simulink library "adeye_lib"  (R2019a)
settings: Solver=VariableStepAuto  StartTime=0.0  StopTime=10.0  RelTol=1e-3
undefined symbols (not defined in the file): AngularVelocity, Clock_, Data, Data_SL_Info, DiscIntNeverNeededParam, Encoding, Encoding_SL_Info, Header, Height, LinearAcceleration, Orientation, Pose, Step, Twist, Width
libraries: robotlib x47, $bdroot x46, simulink_extras x12, dspsrcs4 x6, dspindex x6, robotcorelib x2, aerolibutil x2, PreScanSimulinkLibrary x1
(part 3 of 4)

== system adeye_lib/ROS Send Camera TL ==
  note: Because the image is RGB
  In1 : Inport
  In2 : Inport  Port=2
  In3 : Inport  Port=3
  Enable : EnablePort
  Assignment2 : Assignment  OutputInitialize=Specify size for each dimension in table  DiagnosticForDimensions=Warning  IndexOptions=Starting index (dialog)  Indices=1  OutputSizes=1000
  Blank Message3 : robotlib/Blank Message  messageClass=Message  entityType=sensor_msgs/Image  messageType=sensor_msgs/Image  SampleTime=inf
      settings: SourceProductBaseCode=RO
  Bus Assignment3 : BusAssignment  AssignedSignals=Height,Width,Encoding,Encoding_SL_Info.CurrentLength,Step,Data,Data_SL_Info.CurrentLength,Header.FrameId,Header.FrameId_SL_Info.CurrentLength
  Bus Selector2 : BusSelector  OutputSignals=Header.FrameId
  Constant19 : Constant  Value=uint8(['rgb8'])
  Constant20 : Constant  Value=uint8(['tl_camera'])
  Constant25 : Constant  Value=3  OutDataTypeStr=Inherit: Inherit via back propagation
  Data Type Conversion1 : DataTypeConversion  OutDataTypeStr=uint8
  Ground_1 : Ground
  Ground_2 : Ground
  Ground_3 : Ground
  Math Function{,1..3} (4 alike) : Math  Operator=transpose  SaturateOnIntegerOverflow=on
  Matrix Concatenate : Concatenate  NumInputs=3  Mode=Multidimensional array  ConcatenateDimension=2
  Product : Product  OutDataTypeStr=uint32
  Publish1 : robotlib/Publish  topicSource=Specify your own  topic=sensor/tl/image_raw  messageType=sensor_msgs/Image  messageQueueLength=1
      settings: SourceProductBaseCode=RO
  Reshape{1,17..19} (4 alike) : Reshape
  Terminator_1 : Terminator
  VECTORES : MATLAB Function  TreatAsAtomicUnit=on
  Variable Selector : dspindex/Variable Selector  NumInputs=1  rowsOrCols=Rows  IdxMode=Fixed  Elements=[1]  ZerOneIdxMode=One-based  errmode=Clip Index  FillMode=on  FillValues=0
  Variable Selector1 : dspindex/Variable Selector  NumInputs=1  rowsOrCols=Rows  IdxMode=Fixed  Elements=[1]  ZerOneIdxMode=One-based  errmode=Clip Index  FillMode=on  FillValues=0
  Width : Width
  Width1 : Width
  Width10 : Width  DataType=uint32
  Width5 : Width  DataType=uint32
  Width9 : Width  DataType=uint32
  wires:
  Reshape19/1 -> Matrix Concatenate/3
  Data Type Conversion1/1 -> Width9/1, Bus Assignment3/7
  Math Function/1 -> Variable Selector/1, Reshape17/1
  Constant25/1 -> Product/2
  Width/1 -> Bus Assignment3/2
  Width9/1 -> Bus Assignment3/8
  Bus Selector2/1 -> Assignment2/1  "<FrameId>"
  Product/1 -> Bus Assignment3/6
  Assignment2/1 -> Bus Assignment3/9
  Bus Assignment3/1 -> Publish1/1
  Constant19/1 -> Width5/1, Bus Assignment3/4
  Reshape18/1 -> Matrix Concatenate/2
  Width5/1 -> Bus Assignment3/5
  Reshape17/1 -> Matrix Concatenate/1
  Width10/1 -> Bus Assignment3/10
  Math Function2/1 -> Reshape19/1
  Constant20/1 -> Assignment2/2, Width10/1
  Width1/1 -> Bus Assignment3/3, Product/1
  Math Function1/1 -> Reshape18/1
  Blank Message3/1 -> Bus Selector2/1, Bus Assignment3/1
  In3/1 -> Math Function2/1
  In2/1 -> Math Function1/1
  In1/1 -> Variable Selector1/1, Math Function/1
  Reshape1/1 -> Data Type Conversion1/1
  Matrix Concatenate/1 -> Math Function3/1
  Math Function3/1 -> Reshape1/1
  Variable Selector/1 -> Width/1
  Variable Selector1/1 -> Width1/1
  Ground_1/1 -> VECTORES/1(imgR)
  Ground_2/1 -> VECTORES/2(imgG)
  Ground_3/1 -> VECTORES/3(imgB)
  VECTORES/1(data) -> Terminator_1/1

== system adeye_lib/ROS Send Clock ==
  note: Nanoseconds
  In1 : Inport
  Enable : EnablePort
  Blank Message3 : robotlib/Blank Message  messageClass=Message  entityType=rosgraph_msgs/Clock  messageType=rosgraph_msgs/Clock  SampleTime=inf
      settings: SourceProductBaseCode=RO
  Bus Assignment : BusAssignment  AssignedSignals=Clock_.Sec,Clock_.Nsec
  Constant2 : Constant  Value=1000000000
  Floor : Rounding  Operator=fix
  Product : Product
  Publish3 : robotlib/Publish  topicSource=Specify your own  topic=/clock  messageType=rosgraph_msgs/Clock  messageQueueLength=1
      settings: SourceProductBaseCode=RO
  Subtract : Sum  Inputs=+-
  wires:
  In1/1 -> Subtract/1, Floor/1
  Floor/1 -> Subtract/2, Bus Assignment/2
  Blank Message3/1 -> Bus Assignment/1
  Bus Assignment/1 -> Publish3/1
  Subtract/1 -> Product/1
  Product/1 -> Bus Assignment/3
  Constant2/1 -> Product/2

== system adeye_lib/ROS Send GNSS ==
  In1 : Inport
  Enable : EnablePort
  Add5 : Sum
  Assignment2 : Assignment  OutputInitialize=Specify size for each dimension in table  DiagnosticForDimensions=Warning  IndexOptions=Starting index (dialog)  Indices=1  OutputSizes=1000
  Blank Message4 : robotlib/Blank Message  messageClass=Message  entityType=geometry_msgs/PoseStamped  messageType=geometry_msgs/PoseStamped  SampleTime=inf
      settings: SourceProductBaseCode=RO
  Bus Assignment3 : BusAssignment  AssignedSignals=Header.Seq,Header.FrameId,Header.FrameId_SL_Info.CurrentLength,Header.Stamp.Sec,Header.Stamp.Nsec,Pose.Position.X,Pose.Position.Y,Pose.Position.Z,Pose.Orientation.W,Pose.Orientation.X,Pose.Orientation.Y,Pose.Orientation.Z
  Bus Selector2 : BusSelector  OutputSignals=Header.FrameId
  Clock : Clock
  Constant24 : Constant  OutDataTypeStr=uint32
  Constant25 : Constant  Value=uint8(['map'])
  Demux : Demux  Outputs=7
  Floor : Rounding  Operator=fix
  Memory2 : Memory  InheritSampleTime=on
  Nanoseconds : Constant  Value=1000000000
  Product : Product
  Publish2 : robotlib/Publish  topicSource=Specify your own  topic=/sensor/gnss_pose  messageType=geometry_msgs/PoseStamped  messageQueueLength=1
      settings: SourceProductBaseCode=RO
  Subtract : Sum  Inputs=+-
  Width5 : Width  DataType=uint32
  wires:
  Bus Assignment3/1 -> Publish2/1
  Demux/5 -> Bus Assignment3/11
  Demux/3 -> Bus Assignment3/9
  Product/1 -> Bus Assignment3/6
  Demux/1 -> Bus Assignment3/7
  Add5/1 -> Memory2/1, Bus Assignment3/2
  Clock/1 -> Subtract/1, Floor/1
  In1/1 -> Demux/1  "pose"
  Assignment2/1 -> Bus Assignment3/3
  Bus Selector2/1 -> Assignment2/1  "<FrameId>"
  Constant24/1 -> Add5/2
  Demux/7 -> Bus Assignment3/13
  Demux/6 -> Bus Assignment3/12
  Constant25/1 -> Width5/1, Assignment2/2
  Nanoseconds/1 -> Product/2
  Memory2/1 -> Add5/1
  Blank Message4/1 -> Bus Selector2/1, Bus Assignment3/1
  Floor/1 -> Bus Assignment3/5, Subtract/2
  Width5/1 -> Bus Assignment3/4
  Demux/2 -> Bus Assignment3/8
  Demux/4 -> Bus Assignment3/10
  Subtract/1 -> Product/1

== system adeye_lib/ROS Send Goal ==
  In1 : Inport
  In2 : Inport  Port=2
  In3 : Inport  Port=3
  In4 : Inport  Port=4
  In5 : Inport  Port=5
  In6 : Inport  Port=6
  In7 : Inport  Port=7
  Enable : EnablePort
  Add4 : Sum
  Assignment4 : Assignment  OutputInitialize=Specify size for each dimension in table  DiagnosticForDimensions=Warning  IndexOptions=Starting index (dialog)  Indices=1  OutputSizes=1000
  Blank Message5 : robotlib/Blank Message  messageClass=Message  entityType=geometry_msgs/PoseStamped  messageType=geometry_msgs/PoseStamped  SampleTime=inf
      settings: SourceProductBaseCode=RO
  Bus Assignment4 : BusAssignment  AssignedSignals=Header.Seq,Header.FrameId,Header.FrameId_SL_Info.CurrentLength,Pose.Position.X,Pose.Position.Y,Pose.Position.Z,Pose.Orientation.W,Pose.Orientation.X,Pose.Orientation.Y,Pose.Orientation.Z
  Bus Selector3 : BusSelector  OutputSignals=Header.FrameId
  Constant8 : Constant  OutDataTypeStr=uint32
  Constant9 : Constant  Value=uint8(['world'])
  Memory1 : Memory  InheritSampleTime=on
  Publish1 : robotlib/Publish  topicSource=Select from ROS network  topic=/move_base_simple/goal  messageType=geometry_msgs/PoseStamped  messageQueueLength=1
      settings: SourceProductBaseCode=RO
  Width4 : Width  DataType=uint32
  wires:
  Blank Message5/1 -> Bus Selector3/1, Bus Assignment4/1
  Add4/1 -> Bus Assignment4/2, Memory1/1
  Assignment4/1 -> Bus Assignment4/3
  Bus Selector3/1 -> Assignment4/1  "<FrameId>"
  Bus Assignment4/1 -> Publish1/1
  Constant8/1 -> Add4/2
  Constant9/1 -> Assignment4/2, Width4/1
  Memory1/1 -> Add4/1
  Width4/1 -> Bus Assignment4/4
  In1/1 -> Bus Assignment4/5
  In2/1 -> Bus Assignment4/6
  In3/1 -> Bus Assignment4/7
  In4/1 -> Bus Assignment4/8
  In5/1 -> Bus Assignment4/9
  In6/1 -> Bus Assignment4/10
  In7/1 -> Bus Assignment4/11

== system adeye_lib/ROS Send Groud Truth Pose ==
  In1 : Inport
  Enable : EnablePort
  Add5 : Sum
  Assignment2 : Assignment  OutputInitialize=Specify size for each dimension in table  DiagnosticForDimensions=Warning  IndexOptions=Starting index (dialog)  Indices=1  OutputSizes=1000
  Blank Message4 : robotlib/Blank Message  messageClass=Message  entityType=geometry_msgs/PoseStamped  messageType=geometry_msgs/PoseStamped  SampleTime=inf
      settings: SourceProductBaseCode=RO
  Bus Assignment3 : BusAssignment  AssignedSignals=Header.Seq,Header.FrameId,Header.FrameId_SL_Info.CurrentLength,Header.Stamp.Sec,Header.Stamp.Nsec,Pose.Position.X,Pose.Position.Y,Pose.Position.Z,Pose.Orientation.W,Pose.Orientation.X,Pose.Orientation.Y,Pose.Orientation.Z
  Bus Selector2 : BusSelector  OutputSignals=Header.FrameId
  Clock : Clock
  Constant24 : Constant  OutDataTypeStr=uint32
  Constant25 : Constant  Value=uint8(['map'])
  Demux : Demux  Outputs=7
  Floor : Rounding  Operator=fix
  Memory2 : Memory  InheritSampleTime=on
  Nanoseconds : Constant  Value=1000000000
  Product : Product
  Publish2 : robotlib/Publish  topicSource=Specify your own  topic=/ground_truth_pose  messageType=geometry_msgs/PoseStamped  messageQueueLength=1
      settings: SourceProductBaseCode=RO
  Subtract : Sum  Inputs=+-
  Width5 : Width  DataType=uint32
  wires:
  Constant25/1 -> Width5/1, Assignment2/2
  Clock/1 -> Subtract/1, Floor/1
  Nanoseconds/1 -> Product/2
  Floor/1 -> Bus Assignment3/5, Subtract/2
  Assignment2/1 -> Bus Assignment3/3
  Bus Assignment3/1 -> Publish2/1
  Blank Message4/1 -> Bus Selector2/1, Bus Assignment3/1
  Demux/4 -> Bus Assignment3/10
  Demux/7 -> Bus Assignment3/13
  Demux/5 -> Bus Assignment3/11
  Width5/1 -> Bus Assignment3/4
  Demux/6 -> Bus Assignment3/12
  Demux/2 -> Bus Assignment3/8
  Product/1 -> Bus Assignment3/6
  In1/1 -> Demux/1  "pose"
  Constant24/1 -> Add5/2
  Bus Selector2/1 -> Assignment2/1  "<FrameId>"
  Add5/1 -> Memory2/1, Bus Assignment3/2
  Subtract/1 -> Product/1
  Memory2/1 -> Add5/1
  Demux/1 -> Bus Assignment3/7
  Demux/3 -> Bus Assignment3/9

== system adeye_lib/ROS Send IMU ==
  In1 : Inport
  In2 : Inport  Port=2
  In3 : Inport  Port=3
  Yaw rate [deg/s] : Inport  Port=4
  Velocity [m/s] : Inport  Port=5
  Enable : EnablePort
  Add5 : Sum
  Assignment2 : Assignment  OutputInitialize=Specify size for each dimension in table  DiagnosticForDimensions=Warning  IndexOptions=Starting index (dialog)  Indices=1  OutputSizes=1000
  Blank Message9 : robotlib/Blank Message  messageClass=Message  entityType=sensor_msgs/Imu  messageType=sensor_msgs/Imu  SampleTime=inf
      settings: SourceProductBaseCode=RO
  Bus Assignment7 : BusAssignment  AssignedSignals=Orientation.W,Orientation.X,Orientation.Y,Orientation.Z,AngularVelocity.Z,LinearAcceleration.X,LinearAcceleration.Z,Header.Seq,Header.FrameId,Header.FrameId_SL_Info.CurrentLength
  Bus Selector2 : BusSelector  OutputSignals=Header.FrameId
  Constant : Constant  Value=-9.82
  Constant1 : Constant  Value=-1
  Constant24 : Constant  OutDataTypeStr=uint32
  Constant25 : Constant  Value=uint8(['velodyne'])
  Coordinate Transformation Conversion : robotcorelib/Coordinate Transformation Conversion  InputRepresentation=Euler Angles  InputEulerSequence=XYZ  ShowTrVecInputPort=on  OutputRepresentation=Quaternion  OutputEulerSequence=ZYX  ShowTrVecOutputPort=on  SimulateUsing=Interpreted execution
      settings: SourceProductBaseCode=RO
  Degrees to Radians{1..4} (4 alike) : simulink_extras/Transformations/Degrees to Radians
  Demux : Demux
  Derivative : Derivative
  Memory2 : Memory  InheritSampleTime=on
  Product : Product
  Publish6 : robotlib/Publish  topicSource=Select from ROS network  topic=/imu_raw  messageType=sensor_msgs/Imu  messageQueueLength=1
      settings: SourceProductBaseCode=RO
  Vector Concatenate2 : Concatenate  NumInputs=3
  Width5 : Width  DataType=uint32
  wires:
  Product/1 -> Bus Assignment7/7
  Constant1/1 -> Product/2
  In3/1 -> Degrees to Radians3/1  "Rotational Z [deg]"
  In2/1 -> Degrees to Radians2/1  "Rotational Y [deg]"
  In1/1 -> Degrees to Radians1/1  "Rotational X [deg]"
  Constant/1 -> Bus Assignment7/8
  Velocity [m/s]/1 -> Derivative/1  "Velocity [m/s]"
  Yaw rate [deg/s]/1 -> Degrees to Radians4/1  "Yaw rate [m/s]"
  Demux/4 -> Bus Assignment7/5
  Demux/1 -> Bus Assignment7/2
  Coordinate Transformation Conversion/1 -> Demux/1
  Demux/3 -> Bus Assignment7/4
  Vector Concatenate2/1 -> Coordinate Transformation Conversion/1
  Degrees to Radians3/1 -> Vector Concatenate2/3
  Demux/2 -> Bus Assignment7/3
  Degrees to Radians2/1 -> Vector Concatenate2/2
  Derivative/1 -> Product/1
  Assignment2/1 -> Bus Assignment7/10
  Degrees to Radians4/1 -> Bus Assignment7/6
  Memory2/1 -> Add5/1
  Bus Assignment7/1 -> Publish6/1
  Add5/1 -> Bus Assignment7/9, Memory2/1
  Width5/1 -> Bus Assignment7/11
  Blank Message9/1 -> Bus Assignment7/1, Bus Selector2/1
  Bus Selector2/1 -> Assignment2/1  "<FrameId>"
  Constant25/1 -> Width5/1, Assignment2/2
  Constant24/1 -> Add5/2
  Degrees to Radians1/1 -> Vector Concatenate2/1

== system adeye_lib/ROS Send Lidar ==
  In1 : Inport
  In5 : Inport  Port=2
  In9 : Inport  Port=3
  In13 : Inport  Port=4
  Enable : EnablePort
  Blank Message3 : robotlib/Blank Message  messageClass=Message  entityType=std_msgs/Float32MultiArray  messageType=std_msgs/Float32MultiArray  SampleTime=inf
      settings: SourceProductBaseCode=RO
  Bus Assignment3 : BusAssignment  AssignedSignals=Data,Data_SL_Info.CurrentLength
  Data Type Conversion2 : DataTypeConversion  OutDataTypeStr=single
  Math Function1 : Math  Operator=transpose  SaturateOnIntegerOverflow=on
  Matrix Concatenate5 : Concatenate  NumInputs=4  Mode=Multidimensional array
  Publish1 : robotlib/Publish  topicSource=Specify your own  topic=/points_raw_float32  messageType=std_msgs/Float32MultiArray  messageQueueLength=1
      settings: SourceProductBaseCode=RO
  Reshape17 : Reshape
  Width5 : Width  DataType=uint32
  wires:
  In13/1 -> Matrix Concatenate5/4
  In9/1 -> Matrix Concatenate5/3
  In5/1 -> Matrix Concatenate5/2
  In1/1 -> Matrix Concatenate5/1
  Math Function1/1 -> Reshape17/1
  Data Type Conversion2/1 -> Bus Assignment3/2, Width5/1
  Blank Message3/1 -> Bus Assignment3/1
  Bus Assignment3/1 -> Publish1/1
  Reshape17/1 -> Data Type Conversion2/1
  Matrix Concatenate5/1 -> Math Function1/1
  Width5/1 -> Bus Assignment3/3

== system adeye_lib/ROS Send Odometry ==
  In1 : Inport
  In2 : Inport  Port=2
  In3 : Inport  Port=3
  Enable : EnablePort
  Add5 : Sum
  Assignment2 : Assignment  OutputInitialize=Specify size for each dimension in table  DiagnosticForDimensions=Warning  IndexOptions=Starting index (dialog)  Indices=1  OutputSizes=1000
  Blank Message6 : robotlib/Blank Message  messageClass=Message  entityType=nav_msgs/Odometry  messageType=nav_msgs/Odometry  SampleTime=inf
      settings: SourceProductBaseCode=RO
  Bus Assignment5 : BusAssignment  AssignedSignals=Header.Seq,Header.FrameId,Header.FrameId_SL_Info.CurrentLength,ChildFrameId,ChildFrameId_SL_Info.CurrentLength,Pose.Pose.Position.X,Pose.Pose.Position.Y,Pose.Pose.Position.Z,Pose.Pose.Orientation.W,Pose.Pose.Orientation.X,Pose.Pose.Orientation.Y,Pose.Pose.Orientation.Z,Twist.Twist.Linear.X,Twist.Twist.Linear.Y,Twist.Twist.Linear.Z,Twist.Twist.Angular.X,Twist.Twist.Angular.Y,Twist.Twist.Angular.Z
  Bus Selector2 : BusSelector  OutputSignals=Header.FrameId
  Constant{18..21} (4 alike) : Constant  Value=0
  Constant24 : Constant  OutDataTypeStr=uint32
  Constant25 : Constant  Value=uint8(['/base_link'])
  Degrees to Radians3 : simulink_extras/Transformations/Degrees to Radians
  Demux : Demux  Outputs=7
  Memory2 : Memory  InheritSampleTime=on
  Publish4 : robotlib/Publish  topicSource=Specify your own  topic=/vehicle/odom  messageType=nav_msgs/Odometry  messageQueueLength=1
      settings: SourceProductBaseCode=RO
  Width5 : Width  DataType=uint32
  wires:
  Constant25/1 -> Assignment2/2, Width5/1
  Assignment2/1 -> Bus Assignment5/5, Bus Assignment5/3
  Memory2/1 -> Add5/1
  Constant24/1 -> Add5/2
  Width5/1 -> Bus Assignment5/6, Bus Assignment5/4
  Bus Selector2/1 -> Assignment2/1  "<FrameId>"
  Add5/1 -> Bus Assignment5/2, Memory2/1
  Blank Message6/1 -> Bus Selector2/1, Bus Assignment5/1
  Bus Assignment5/1 -> Publish4/1
  In3/1 -> Degrees to Radians3/1
  Constant18/1 -> Bus Assignment5/15
  Degrees to Radians3/1 -> Bus Assignment5/19
  Constant20/1 -> Bus Assignment5/17
  Constant19/1 -> Bus Assignment5/16
  Constant21/1 -> Bus Assignment5/18
  In2/1 -> Bus Assignment5/14
  Demux/3 -> Bus Assignment5/9
  Demux/2 -> Bus Assignment5/8
  Demux/7 -> Bus Assignment5/13
  Demux/6 -> Bus Assignment5/12
  In1/1 -> Demux/1
  Demux/4 -> Bus Assignment5/10
  Demux/5 -> Bus Assignment5/11
  Demux/1 -> Bus Assignment5/7

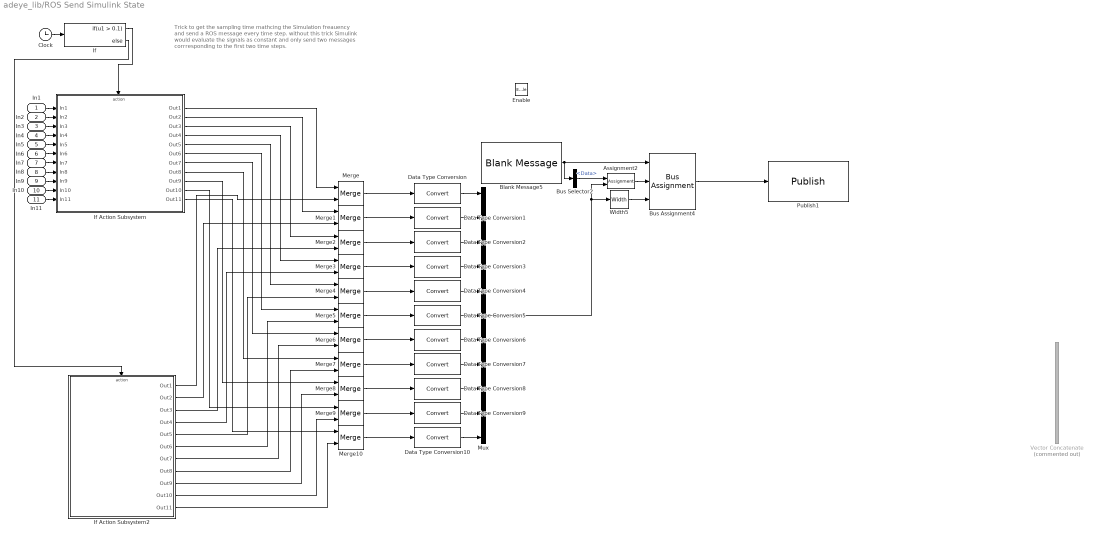
== system adeye_lib/ROS Send Simulink State ==
  note: Trick to get the sampling time mathcing the Simulation freauency and send a ROS message every time step. without this trick Simulink would evaluate the signals as constant and only send two messages corrresponding to the first two time steps.
  In1 : Inport
  In2 : Inport  Port=2
  In3 : Inport  Port=3
  In4 : Inport  Port=4
  In5 : Inport  Port=5
  In6 : Inport  Port=6
  In7 : Inport  Port=7
  In8 : Inport  Port=8
  In9 : Inport  Port=9
  In10 : Inport  Port=10
  In11 : Inport  Port=11
  Enable : EnablePort
  Assignment2 : Assignment  OutputInitialize=Specify size for each dimension in table  DiagnosticForDimensions=Warning  IndexOptions=Starting index (dialog)  Indices=1  OutputSizes=1000
  Blank Message5 : robotlib/Blank Message  messageClass=Message  entityType=std_msgs/Int32MultiArray  messageType=std_msgs/Int32MultiArray  SampleTime=inf
      settings: SourceProductBaseCode=RO
  Bus Assignment4 : BusAssignment  AssignedSignals=Data,Data_SL_Info.CurrentLength
  Bus Selector2 : BusSelector  OutputSignals=Data
  Clock : Clock
  Data Type Conversion{,1..10} (11 alike) : DataTypeConversion
  If : If  IfExpression=u1 > 0.1
  If Action Subsystem : Subsystem  TreatAsAtomicUnit=on
  If Action Subsystem2 : Subsystem  TreatAsAtomicUnit=on
  Merge{,1..10} (11 alike) : Merge
  Mux : Mux  Inputs=11
  Publish1 : robotlib/Publish  topicSource=Specify your own  topic=/Features_state  messageType=std_msgs/Int32MultiArray  messageQueueLength=1
      settings: SourceProductBaseCode=RO
  Vector Concatenate : Concatenate  Commented=on  NumInputs=10
  Width5 : Width  DataType=uint32
  wires:
  Assignment2/1 -> Bus Assignment4/2
  Blank Message5/1 -> Bus Assignment4/1, Bus Selector2/1
  Bus Selector2/1 -> Assignment2/1  "<Data>"
  Width5/1 -> Bus Assignment4/3
  Bus Assignment4/1 -> Publish1/1
  Mux/1 -> Width5/1, Assignment2/2
  In11/1 -> If Action Subsystem/11(In11)
  In10/1 -> If Action Subsystem/10(In10)
  In9/1 -> If Action Subsystem/9(In9)
  In8/1 -> If Action Subsystem/8(In8)
  In7/1 -> If Action Subsystem/7(In7)
  In6/1 -> If Action Subsystem/6(In6)
  In5/1 -> If Action Subsystem/5(In5)
  In4/1 -> If Action Subsystem/4(In4)
  In3/1 -> If Action Subsystem/3(In3)
  In2/1 -> If Action Subsystem/2(In2)
  In1/1 -> If Action Subsystem/1(In1)
  Merge/1 -> Data Type Conversion/1
  Merge1/1 -> Data Type Conversion1/1
  Merge2/1 -> Data Type Conversion2/1
  Merge3/1 -> Data Type Conversion3/1
  Merge4/1 -> Data Type Conversion4/1
  Merge5/1 -> Data Type Conversion5/1
  Merge6/1 -> Data Type Conversion6/1
  Merge7/1 -> Data Type Conversion7/1
  Merge8/1 -> Data Type Conversion8/1
  Merge9/1 -> Data Type Conversion9/1
  Merge10/1 -> Data Type Conversion10/1
  If/2 -> If Action Subsystem2/Action
  If/1 -> If Action Subsystem/Action
  Clock/1 -> If/1
  If Action Subsystem/1(Out1) -> Merge/1
  If Action Subsystem/2(Out2) -> Merge1/1
  If Action Subsystem/3(Out3) -> Merge2/1
  If Action Subsystem/4(Out4) -> Merge3/1
  If Action Subsystem/5(Out5) -> Merge4/1
  If Action Subsystem/6(Out6) -> Merge5/1
  If Action Subsystem/7(Out7) -> Merge6/1
  If Action Subsystem/8(Out8) -> Merge7/1
  If Action Subsystem/9(Out9) -> Merge8/1
  If Action Subsystem/10(Out10) -> Merge9/1
  If Action Subsystem/11(Out11) -> Merge10/1
  If Action Subsystem2/1(Out1) -> Merge/2
  If Action Subsystem2/2(Out2) -> Merge1/2
  If Action Subsystem2/3(Out3) -> Merge2/2
  If Action Subsystem2/4(Out4) -> Merge3/2
  If Action Subsystem2/5(Out5) -> Merge4/2
  If Action Subsystem2/6(Out6) -> Merge5/2
  If Action Subsystem2/7(Out7) -> Merge6/2
  If Action Subsystem2/8(Out8) -> Merge7/2
  If Action Subsystem2/9(Out9) -> Merge8/2
  If Action Subsystem2/10(Out10) -> Merge9/2
  If Action Subsystem2/11(Out11) -> Merge10/2
  Data Type Conversion/1 -> Mux/1
  Data Type Conversion1/1 -> Mux/2
  Data Type Conversion2/1 -> Mux/3
  Data Type Conversion3/1 -> Mux/4
  Data Type Conversion4/1 -> Mux/5
  Data Type Conversion5/1 -> Mux/6
  Data Type Conversion6/1 -> Mux/7
  Data Type Conversion7/1 -> Mux/8
  Data Type Conversion8/1 -> Mux/9
  Data Type Conversion9/1 -> Mux/10
  Data Type Conversion10/1 -> Mux/11

== system adeye_lib/ROS Send Switch Command ==
  In1 : Inport
  Enable : EnablePort
  Blank Message3 : robotlib/Blank Message  messageClass=Message  entityType=std_msgs/Int32  messageType=std_msgs/Int32  SampleTime=inf
      settings: SourceProductBaseCode=RO
  Bus Assignment : BusAssignment  AssignedSignals=Data
  Publish3 : robotlib/Publish  topicSource=Specify your own  topic=/switch_command  messageType=std_msgs/Int32  messageQueueLength=1
      settings: SourceProductBaseCode=RO
  wires:
  Blank Message3/1 -> Bus Assignment/1
  Bus Assignment/1 -> Publish3/1
  In1/1 -> Bus Assignment/2

== system adeye_lib/ROS Send Velocity ==
  In1 : Inport
  In2 : Inport  Port=2
  Enable : EnablePort
  Add5 : Sum
  Assignment2 : Assignment  OutputInitialize=Specify size for each dimension in table  DiagnosticForDimensions=Warning  IndexOptions=Starting index (dialog)  Indices=1  OutputSizes=1000
  Blank Message6 : robotlib/Blank Message  messageClass=Message  entityType=geometry_msgs/TwistStamped  messageType=geometry_msgs/TwistStamped  SampleTime=inf
      settings: SourceProductBaseCode=RO
  Bus Assignment5 : BusAssignment  AssignedSignals=Header.Seq,Header.FrameId,Header.FrameId_SL_Info.CurrentLength,Twist.Linear.X,Twist.Linear.Y,Twist.Linear.Z,Twist.Angular.X,Twist.Angular.Y,Twist.Angular.Z
  Bus Selector2 : BusSelector  OutputSignals=Header.FrameId
  Constant{18..21} (4 alike) : Constant  Value=0
  Constant24 : Constant  OutDataTypeStr=uint32
  Constant25 : Constant  Value=uint8(['/base_link'])
  Degrees to Radians3 : simulink_extras/Transformations/Degrees to Radians
  Memory2 : Memory  InheritSampleTime=on
  Publish4 : robotlib/Publish  topicSource=Select from ROS network  topic=/current_velocity  messageType=geometry_msgs/TwistStamped  messageQueueLength=1
      settings: SourceProductBaseCode=RO
  Width5 : Width  DataType=uint32
  wires:
  Constant25/1 -> Assignment2/2, Width5/1
  Assignment2/1 -> Bus Assignment5/3
  Memory2/1 -> Add5/1
  Degrees to Radians3/1 -> Bus Assignment5/10
  Constant19/1 -> Bus Assignment5/7
  Constant24/1 -> Add5/2
  Width5/1 -> Bus Assignment5/4
  Constant20/1 -> Bus Assignment5/8
  Bus Selector2/1 -> Assignment2/1  "<FrameId>"
  Add5/1 -> Bus Assignment5/2, Memory2/1
  Constant18/1 -> Bus Assignment5/6
  Blank Message6/1 -> Bus Selector2/1, Bus Assignment5/1
  Constant21/1 -> Bus Assignment5/9
  Bus Assignment5/1 -> Publish4/1
  In1/1 -> Bus Assignment5/5
  In2/1 -> Degrees to Radians3/1

== system adeye_lib/ROS Stop Experiment ==
  Bus Selector : BusSelector  OutputSignals=Data
  Stop Simulation : Stop
  Subscribe : robotlib/Subscribe  topicSource=Specify your own  topic=/simulink/stop_experiment  messageType=std_msgs/Bool  sampleTime=-1  messageQueueLength=1
      settings: SourceProductBaseCode=RO
  Terminator : Terminator
  wires:
  Subscribe/2 -> Bus Selector/1
  Bus Selector/1 -> Stop Simulation/1  "<Data>"
  Subscribe/1 -> Terminator/1

== system adeye_lib/ROS send RCV states ==
  In1 : Inport
  In2 : Inport  Port=2
  In3 : Inport  Port=3
  Blank Message : robotlib/Blank Message  messageClass=Message  entityType=std_msgs/Bool  messageType=std_msgs/Bool  SampleTime=inf
      settings: SourceProductBaseCode=RO
  Blank Message1 : robotlib/Blank Message  messageClass=Message  entityType=std_msgs/Bool  messageType=std_msgs/Bool  SampleTime=inf
      settings: SourceProductBaseCode=RO
  Blank Message2 : robotlib/Blank Message  messageClass=Message  entityType=std_msgs/Bool  messageType=std_msgs/Bool  SampleTime=inf
      settings: SourceProductBaseCode=RO
  Bus Assignment : BusAssignment  AssignedSignals=Data
  Bus Assignment1 : BusAssignment  AssignedSignals=Data
  Bus Assignment2 : BusAssignment  AssignedSignals=Data
  Publish : robotlib/Publish  topicSource=Select from ROS network  topic=/initial_checks  messageType=std_msgs/Bool  messageQueueLength=1
      settings: SourceProductBaseCode=RO
  Publish1 : robotlib/Publish  topicSource=Select from ROS network  topic=/activation_request  messageType=std_msgs/Bool  messageQueueLength=1
      settings: SourceProductBaseCode=RO
  Publish2 : robotlib/Publish  topicSource=Select from ROS network  topic=/fault  messageType=std_msgs/Bool  messageQueueLength=1
      settings: SourceProductBaseCode=RO
  wires:
  In3/1 -> Bus Assignment2/2
  Bus Assignment2/1 -> Publish2/1
  Blank Message1/1 -> Bus Assignment1/1
  Blank Message2/1 -> Bus Assignment2/1
  Bus Assignment1/1 -> Publish1/1
  Blank Message/1 -> Bus Assignment/1
  Bus Assignment/1 -> Publish/1
  In2/1 -> Bus Assignment1/2
  In1/1 -> Bus Assignment/2

== system adeye_lib/Subsystem1 ==
  note: For state mode 'Dynamic' positions
      | are not taken into account, as they
      | are computed by integrating velocity.
      | Click annotation for Help.
  In1 : Inport
  Bus Selector1 : BusSelector  OutputSignals=Twist.Linear.X,Twist.Linear.Y,Twist.Linear.Z,Twist.Angular.X,Twist.Angular.Y,Twist.Angular.Z
  Data Type Conversion{6..11} (6 alike) : DataTypeConversion
  Discrete-Time Integrator4 : DiscreteIntegrator  SampleTime=-1  ICPrevOutput=DiscIntNeverNeededParam  ICPrevScaledInput=DiscIntNeverNeededParam
  Discrete-Time Integrator5 : DiscreteIntegrator  SampleTime=-1  ICPrevOutput=DiscIntNeverNeededParam  ICPrevScaledInput=DiscIntNeverNeededParam
  Discrete-Time Integrator6 : DiscreteIntegrator  SampleTime=-1  ICPrevOutput=DiscIntNeverNeededParam  ICPrevScaledInput=DiscIntNeverNeededParam
  Subscribe1 : robotlib/Subscribe  topicSource=Select from ROS network  topic=/TwistS  messageType=geometry_msgs/TwistStamped  sampleTime=-1  messageQueueLength=1
      settings: SourceProductBaseCode=RO
  Subsystem : Subsystem
  Terminator_4 : Terminator
  Out1 : Outport
  Out2 : Outport  Port=2
  Out3 : Outport  Port=3
  Out4 : Outport  Port=4
  Out5 : Outport  Port=5
  Out6 : Outport  Port=6
  wires:
  Data Type Conversion6/1 -> Subsystem/2(In2)
  Bus Selector1/2 -> Data Type Conversion7/1  "<Y>"
  Bus Selector1/5 -> Data Type Conversion10/1  "<Y>"
  Data Type Conversion11/1 -> Discrete-Time Integrator4/1
  Bus Selector1/6 -> Data Type Conversion11/1  "<Z>"
  Bus Selector1/4 -> Data Type Conversion9/1  "<X>"
  Bus Selector1/1 -> Data Type Conversion6/1  "<X>"
  Data Type Conversion10/1 -> Discrete-Time Integrator5/1
  Subscribe1/1 -> Terminator_4/1
  Data Type Conversion9/1 -> Discrete-Time Integrator6/1
  Bus Selector1/3 -> Data Type Conversion8/1  "<Z>"
  Subscribe1/2 -> Bus Selector1/1
  Discrete-Time Integrator5/1 -> Out5/1
  Data Type Conversion7/1 -> Out2/1
  Discrete-Time Integrator4/1 -> Out6/1
  Data Type Conversion8/1 -> Out3/1
  Subsystem/1(Out1) -> Out1/1
  In1/1 -> Subsystem/1(In1)
  Discrete-Time Integrator6/1 -> Out4/1

== system adeye_lib/frequency_evaluator ==
  note: This was set to 0.999 instead of 1 to have
      | some tolerance the the grater that comparison.
      |
      | In other word, we accept an error of
      | 0.001 period in the greater than
      | comparison.
      |
      | Without this tolerance, issues with floating
      | point precision happen making the greater
      | than produce wrong output
  frequency : Inport
  Add : Sum  Inputs=+-
  Clock2 : Clock
  Constant : Constant  Value=0.999
  Divide : Product  Inputs=*/
  Memory : Memory
  Relational Operator : RelationalOperator  OutDataTypeStr=boolean  RndMeth=Simplest
  Switch : Switch  Criteria=u2 > Threshold
  enable : Outport
  wires:
  Constant/1 -> Divide/1
  frequency/1 -> Divide/2  "frequency"
  Clock2/1 -> Switch/1, Add/1  "current simulation time"
  Switch/1 -> Memory/1
  Memory/1 -> Switch/3, Add/2  "last trigger time"
  Divide/1 -> Relational Operator/2  "period"
  Relational Operator/1 -> Switch/2, enable/1  "trigger"
  Add/1 -> Relational Operator/1  "time since last triger"

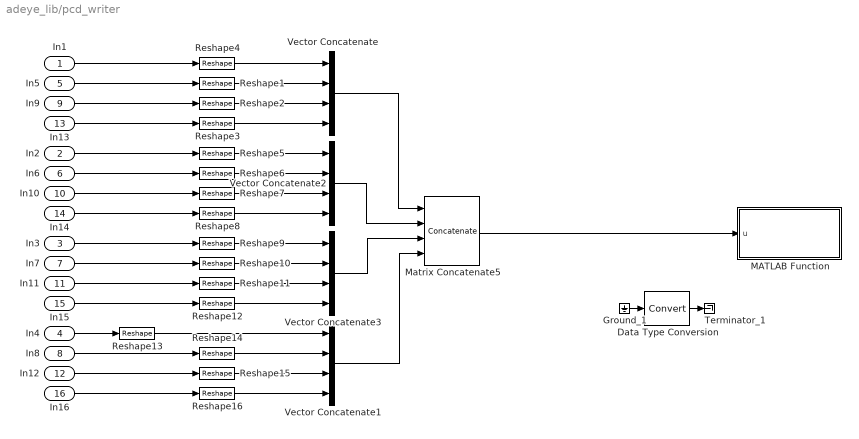
== system adeye_lib/pcd_writer ==
  In1 : Inport
  In2 : Inport  Port=2
  In3 : Inport  Port=3
  In4 : Inport  Port=4
  In5 : Inport  Port=5
  In6 : Inport  Port=6
  In7 : Inport  Port=7
  In8 : Inport  Port=8
  In9 : Inport  Port=9
  In10 : Inport  Port=10
  In11 : Inport  Port=11
  In12 : Inport  Port=12
  In13 : Inport  Port=13
  In14 : Inport  Port=14
  In15 : Inport  Port=15
  In16 : Inport  Port=16
  Data Type Conversion : DataTypeConversion
  Ground_1 : Ground
  MATLAB Function : MATLAB Function  TreatAsAtomicUnit=on
  Matrix Concatenate5 : Concatenate  NumInputs=4  Mode=Multidimensional array  ConcatenateDimension=2
  Reshape{1..16} (16 alike) : Reshape
  Terminator_1 : Terminator
  Vector Concatenate{,1..3} (4 alike) : Concatenate  NumInputs=4
  wires:
  Data Type Conversion/1 -> Terminator_1/1
  Ground_1/1 -> Data Type Conversion/1
  Matrix Concatenate5/1 -> MATLAB Function/1(u)
  Vector Concatenate1/1 -> Matrix Concatenate5/4
  Vector Concatenate3/1 -> Matrix Concatenate5/3
  Vector Concatenate2/1 -> Matrix Concatenate5/2
  Vector Concatenate/1 -> Matrix Concatenate5/1
  Reshape16/1 -> Vector Concatenate1/4
  Reshape15/1 -> Vector Concatenate1/3
  Reshape14/1 -> Vector Concatenate1/2
  Reshape13/1 -> Vector Concatenate1/1
  Reshape12/1 -> Vector Concatenate3/4
  Reshape11/1 -> Vector Concatenate3/3
  Reshape10/1 -> Vector Concatenate3/2
  Reshape9/1 -> Vector Concatenate3/1
  Reshape8/1 -> Vector Concatenate2/4
  Reshape7/1 -> Vector Concatenate2/3
  Reshape6/1 -> Vector Concatenate2/2
  Reshape5/1 -> Vector Concatenate2/1
  Reshape3/1 -> Vector Concatenate/4
  Reshape2/1 -> Vector Concatenate/3
  Reshape1/1 -> Vector Concatenate/2
  Reshape4/1 -> Vector Concatenate/1
  In16/1 -> Reshape16/1
  In15/1 -> Reshape12/1
  In14/1 -> Reshape8/1
  In13/1 -> Reshape3/1
  In12/1 -> Reshape15/1
  In11/1 -> Reshape11/1
  In10/1 -> Reshape7/1
  In9/1 -> Reshape2/1
  In8/1 -> Reshape14/1
  In7/1 -> Reshape10/1
  In6/1 -> Reshape6/1
  In5/1 -> Reshape1/1
  In4/1 -> Reshape13/1
  In3/1 -> Reshape9/1
  In2/1 -> Reshape5/1
  In1/1 -> Reshape4/1

== system adeye_lib/radarDetections ==
  In1 : Inport
  In2 : Inport  Port=2
  In3 : Inport  Port=3
  In4 : Inport  Port=4
  Enable : EnablePort
  Assignment2 : Assignment  OutputInitialize=Specify size for each dimension in table  DiagnosticForDimensions=Warning  IndexOptions=Starting index (dialog)  Indices=1  OutputSizes=1000
  Blank Message3 : robotlib/Blank Message  messageClass=Message  entityType=std_msgs/Float32MultiArray  messageType=std_msgs/Float32MultiArray  SampleTime=inf
      settings: SourceProductBaseCode=RO
  Bus Assignment3 : BusAssignment  AssignedSignals=Data,Data_SL_Info.CurrentLength
  Bus Selector2 : BusSelector  OutputSignals=Data
  Constant : Constant
  Data Type Conversion2 : DataTypeConversion  OutDataTypeStr=single
  Degrees to Radians : simulink_extras/Transformations/Degrees to Radians
  Degrees to Radians1 : simulink_extras/Transformations/Degrees to Radians
  Display3 : Display
  Math Function1 : Math  Operator=transpose  SaturateOnIntegerOverflow=on
  Matrix Concatenate5 : Concatenate  NumInputs=3  Mode=Multidimensional array  ConcatenateDimension=2
  Product : Product
  Product1 : Product
  Product2 : Product
  Publish1 : robotlib/Publish  topicSource=Specify your own  topic=/radarDetections  messageType=std_msgs/Float32MultiArray  messageQueueLength=1
      settings: SourceProductBaseCode=RO
  Relational Operator : RelationalOperator  Operator===  OutDataTypeStr=boolean  RndMeth=Simplest
  Reshape{1..4,17} (5 alike) : Reshape
  Spherical to cartesian : Subsystem
  Width5 : Width  DataType=uint32
  wires:
  Constant/1 -> Relational Operator/2
  Spherical to cartesian/3(Out3) -> Matrix Concatenate5/3
  In4/1 -> Reshape4/1
  Product2/1 -> Spherical to cartesian/3(In3)
  Bus Assignment3/1 -> Publish1/1
  Blank Message3/1 -> Bus Assignment3/1, Bus Selector2/1
  Matrix Concatenate5/1 -> Math Function1/1
  In1/1 -> Reshape2/1
  Spherical to cartesian/1(Out1) -> Matrix Concatenate5/1
  Width5/1 -> Bus Assignment3/3
  Reshape2/1 -> Product/1
  In3/1 -> Degrees to Radians1/1
  Reshape4/1 -> Relational Operator/1
  In2/1 -> Degrees to Radians/1
  Relational Operator/1 -> Product2/2, Product1/2, Product/2
  Reshape17/1 -> Data Type Conversion2/1, Display3/1
  Reshape1/1 -> Product1/1
  Assignment2/1 -> Bus Assignment3/2
  Data Type Conversion2/1 -> Assignment2/2, Width5/1
  Degrees to Radians1/1 -> Reshape3/1
  Reshape3/1 -> Product2/1
  Spherical to cartesian/2(Out2) -> Matrix Concatenate5/2
  Degrees to Radians/1 -> Reshape1/1
  Product/1 -> Spherical to cartesian/1(In1)
  Bus Selector2/1 -> Assignment2/1  "<Data>"
  Math Function1/1 -> Reshape17/1
  Product1/1 -> Spherical to cartesian/2(In2)

== system adeye_lib/Dynamics_Empty/MuxState ==
  note: For state mode 'Dynamic' positions
      | are not taken into account, as they
      | are computed by integrating velocity.
      | Click annotation for Help.
  note: AnglesVEHICLE
      | wrtGLOB
  note: mode: Dynamics
      | VelVEHICLE
      | wrt VEH
  note: mode: Positioning
  note: mode: Dynamics
  x [m] : Inport  SampleTime=TimeStep
  y [m] : Inport  Port=2  SampleTime=TimeStep
  z [m] : Inport  Port=3  SampleTime=TimeStep
  dx [m/s] : Inport  Port=4  SampleTime=TimeStep
  dy [m/s] : Inport  Port=5  SampleTime=TimeStep
  dz [m/s] : Inport  Port=6  SampleTime=TimeStep
  R [rad] : Inport  Port=7  SampleTime=TimeStep
  P [rad] : Inport  Port=8  SampleTime=TimeStep
  Y [rad] : Inport  Port=9  SampleTime=TimeStep
  Constant : Constant  DisableCoverage=on  Value=positioningmode
  Discrete-Time Integrator : DiscreteIntegrator  SampleTime=TimeStep  ICPrevOutput=DiscIntNeverNeededParam  ICPrevScaledInput=DiscIntNeverNeededParam
  Ground : Ground
  Ground1 : Ground
  Mux1 : Mux  Inputs=[3 3]
  Mux2 : Mux  Inputs=3
  Mux3 : Mux  Inputs=3
  Mux4 : Mux  Inputs=3
  Mux5 : Mux  Inputs=[3 3]
  Mux6 : Mux  Inputs=[6 3]
  Switch : Switch  Threshold=0.5
  Transformation_BODY2GLOBAL : PreScanSimulinkLibrary/Simple_Vehicle_Dynamics/Chassis/MuxDynState/Transformation_BODY2GLOBAL  SystemSampleTime=-1
  mux3 : Mux  Inputs=3
  state : Outport
  wires:
  Discrete-Time Integrator/1 -> Mux5/1  "PosVEH wrt  GLOB"
  Mux2/1 -> Transformation_BODY2GLOBAL/1, Mux1/2
  Ground/1 -> mux3/1  "roll"
  mux3/1 -> Transformation_BODY2GLOBAL/2
  Transformation_BODY2GLOBAL/1 -> Mux5/2, Discrete-Time Integrator/1  "VelVEH wrt  GLOB"
  Mux3/1 -> Mux6/2
  Y [rad]/1 -> Mux3/3, mux3/3  "yaw"
  Ground1/1 -> mux3/2  "pitch"
  x [m]/1 -> Mux4/1
  y [m]/1 -> Mux4/2
  z [m]/1 -> Mux4/3
  dx [m/s]/1 -> Mux2/1
  dy [m/s]/1 -> Mux2/2
  dz [m/s]/1 -> Mux2/3
  R [rad]/1 -> Mux3/1
  P [rad]/1 -> Mux3/2
  Switch/1 -> Mux6/1  "PosVeh wrt  GLOB"
  Mux1/1 -> Switch/1
  Mux5/1 -> Switch/3
  Mux4/1 -> Mux1/1
  Mux6/1 -> state/1
  Constant/1 -> Switch/2

== system adeye_lib/Fault Injection Camera/If Action Subsystem ==
  In1 : Inport
  In2 : Inport  Port=2
  In3 : Inport  Port=3
  Action Port : ActionPort
  Out1 : Outport
  Out2 : Outport  Port=2
  Out3 : Outport  Port=3
  wires:
  In3/1 -> Out3/1
  In2/1 -> Out2/1
  In1/1 -> Out1/1

== system adeye_lib/Fault Injection Camera/If Action Subsystem1 ==
  note: Those are placeholders for
      |  the patch dimensions inputs.
      | Using them reauires a
      | reimplementation of the
      | patch fault injection.
  image_R : Inport
  image_G : Inport  Port=2
  image_B : Inport  Port=3
  start_x : Inport  Port=4
  start_y : Inport  Port=5
  size_x : Inport  Port=6
  size_y : Inport  Port=7
  patch_R : Inport  Port=8
  patch_G : Inport  Port=9
  patch_B : Inport  Port=10
  Action Port : ActionPort
  Assignment1 : Assignment  NumberOfDimensions=2  DiagnosticForDimensions=Warning  IndexOptions=Starting index (port),Starting index (port)  Indices=1,1  OutputSizes=1000,1
  Assignment2 : Assignment  NumberOfDimensions=2  DiagnosticForDimensions=Warning  IndexOptions=Starting index (port),Starting index (port)  Indices=1,1  OutputSizes=1000,1
  Assignment3 : Assignment  NumberOfDimensions=2  DiagnosticForDimensions=Warning  IndexOptions=Starting index (port),Starting index (port)  Indices=1,1  OutputSizes=1000,1
  Constant1 : Constant  Value=ones(x,y)  OutDataTypeStr=uint8
  Constant2 : Constant  Value=ones(x,y)  OutDataTypeStr=uint8
  Constant4 : Constant  Value=ones(x,y)  OutDataTypeStr=uint8
  Data Type Conversion{,1..5} (6 alike) : DataTypeConversion
  Product : Product  InputSameDT=on
  Product1 : Product  InputSameDT=on
  Product2 : Product  InputSameDT=on
  Terminator : Terminator
  Terminator1 : Terminator
  Output_image_R : Outport
  Output_image_G : Outport  Port=2
  Output_image_B : Outport  Port=3
  wires:
  start_y/1 -> Assignment3/4, Assignment1/4, Assignment2/4
  image_R/1 -> Assignment2/1
  image_B/1 -> Assignment3/1
  Assignment3/1 -> Output_image_B/1
  Assignment2/1 -> Output_image_R/1
  Assignment1/1 -> Output_image_G/1
  image_G/1 -> Assignment1/1
  start_x/1 -> Assignment2/3, Assignment1/3, Assignment3/3
  size_y/1 -> Terminator1/1
  size_x/1 -> Terminator/1
  Constant4/1 -> Product/1
  patch_R/1 -> Data Type Conversion2/1
  Constant1/1 -> Product1/1
  patch_G/1 -> Data Type Conversion1/1
  Constant2/1 -> Product2/1
  patch_B/1 -> Data Type Conversion/1
  Data Type Conversion/1 -> Product2/2
  Data Type Conversion1/1 -> Product1/2
  Data Type Conversion2/1 -> Product/2
  Product2/1 -> Data Type Conversion3/1
  Data Type Conversion3/1 -> Assignment3/2
  Data Type Conversion5/1 -> Assignment2/2
  Data Type Conversion4/1 -> Assignment1/2
  Product1/1 -> Data Type Conversion4/1
  Product/1 -> Data Type Conversion5/1

== system adeye_lib/Fault Injection GNSS/If Action Subsystem ==
  In1 : Inport
  Action Port : ActionPort
  Out1 : Outport
  wires:
  In1/1 -> Out1/1

== system adeye_lib/Fault Injection GNSS/If Action Subsystem1 ==
  In1 : Inport
  noise_variance : Inport  Port=2
  Action Port : ActionPort
  Demux : Demux  Outputs=7
  Mux1 : Mux  Inputs=7
  Product1 : Product
  Product2 : Product
  Product4 : Product
  Random Source1 : dspsrcs4/Random Source  SrcType=Gaussian  NormMethod=Ziggurat  CltLength=12  MinVal=0  MaxVal=1  MeanVal=0  VarVal=1  RepMode=Not repeatable  rawSeed=1  IsInherit=off  SampMode=Discrete  SampTime=-1  SampFrame=1  DataType=Single  OutComplex=Real  OutputFrames=off
  Random Source2 : dspsrcs4/Random Source  SrcType=Gaussian  NormMethod=Ziggurat  CltLength=12  MinVal=0  MaxVal=1  MeanVal=0  VarVal=1  RepMode=Not repeatable  rawSeed=1  IsInherit=off  SampMode=Discrete  SampTime=-1  SampFrame=1  DataType=Single  OutComplex=Real  OutputFrames=off
  Random Source3 : dspsrcs4/Random Source  SrcType=Gaussian  NormMethod=Ziggurat  CltLength=12  MinVal=0  MaxVal=1  MeanVal=0  VarVal=1  RepMode=Not repeatable  rawSeed=1  IsInherit=off  SampMode=Discrete  SampTime=-1  SampFrame=1  DataType=Single  OutComplex=Real  OutputFrames=off
  Signal Conversion{1..4} (4 alike) : SignalConversion  OverrideOpt=off
  Sqrt : Sqrt  SaturateOnIntegerOverflow=on
  Subtract : Sum
  Subtract1 : Sum
  Subtract2 : Sum
  Out1 : Outport
  wires:
  Demux/1 -> Subtract/2
  Subtract/1 -> Mux1/1
  In1/1 -> Demux/1
  Demux/2 -> Subtract1/2
  Subtract1/1 -> Mux1/2
  Demux/3 -> Subtract2/2
  Subtract2/1 -> Mux1/3
  Demux/5 -> Signal Conversion1/1
  Demux/6 -> Signal Conversion2/1
  Demux/7 -> Signal Conversion3/1
  Mux1/1 -> Out1/1
  Signal Conversion3/1 -> Mux1/7
  Signal Conversion2/1 -> Mux1/6
  Signal Conversion1/1 -> Mux1/5
  Demux/4 -> Signal Conversion4/1
  Signal Conversion4/1 -> Mux1/4
  noise_variance/1 -> Sqrt/1
  Product4/1 -> Subtract2/1
  Random Source3/1 -> Product4/2
  Product2/1 -> Subtract1/1
  Random Source2/1 -> Product2/2
  Product1/1 -> Subtract/1
  Random Source1/1 -> Product1/2
  Sqrt/1 -> Product4/1, Product2/1, Product1/1

== system adeye_lib/Fault Injection Lidar/If Action Subsystem ==
  Range : Inport
  Theta : Inport  Port=2
  Phi : Inport  Port=3
  Intensity : Inport  Port=4
  Action Port : ActionPort  ActionPortLabel=else
  Out1 : Outport
  Out2 : Outport  Port=2
  Out3 : Outport  Port=3
  Out4 : Outport  Port=4
  wires:
  Range/1 -> Out1/1
  Theta/1 -> Out2/1
  Phi/1 -> Out3/1
  Intensity/1 -> Out4/1

== system adeye_lib/Fault Injection Lidar/If Action Subsystem1 ==
  Range : Inport
  Theta : Inport  Port=2
  Phi : Inport  Port=3
  Intensity : Inport  Port=4
  range_variance : Inport  Port=5
  theta_variance : Inport  Port=6
  Action Port : ActionPort  ActionPortLabel=elseif(u1 > 0)
  Data Type Conversion : DataTypeConversion
  Data Type Conversion1 : DataTypeConversion
  Product{,1..3} (4 alike) : Product
  Random Source1 : dspsrcs4/Random Source  SrcType=Gaussian  NormMethod=Ziggurat  CltLength=12  MinVal=0  MaxVal=1  MeanVal=0  VarVal=1  RepMode=Not repeatable  rawSeed=1  IsInherit=off  SampMode=Discrete  SampTime=1/(f*p)  SampFrame=p  DataType=Single  OutComplex=Real  OutputFrames=off
  Random Source2 : dspsrcs4/Random Source  SrcType=Gaussian  NormMethod=Ziggurat  CltLength=12  MinVal=0  MaxVal=1  MeanVal=0  VarVal=1  RepMode=Not repeatable  rawSeed=1  IsInherit=off  SampMode=Discrete  SampTime=1/(f*p)  SampFrame=p  DataType=Single  OutComplex=Real  OutputFrames=off
  Sqrt : Sqrt  SaturateOnIntegerOverflow=on
  Sqrt1 : Sqrt  SaturateOnIntegerOverflow=on
  Subtract : Sum
  Subtract1 : Sum
  Out1 : Outport
  Out2 : Outport  Port=2
  Out3 : Outport  Port=3
  Out4 : Outport  Port=4
  wires:
  Phi/1 -> Out3/1
  Intensity/1 -> Out4/1
  Subtract/1 -> Out1/1
  Subtract1/1 -> Out2/1
  Range/1 -> Subtract/2, Product/2
  Theta/1 -> Subtract1/2, Product1/2
  Random Source2/1 -> Product2/2
  Product3/1 -> Product/1
  Product2/1 -> Product1/1
  Random Source1/1 -> Product3/2
  theta_variance/1 -> Sqrt1/1
  range_variance/1 -> Sqrt/1
  Sqrt/1 -> Product3/1
  Sqrt1/1 -> Product2/1
  Data Type Conversion/1 -> Subtract/1
  Product/1 -> Data Type Conversion/1
  Data Type Conversion1/1 -> Subtract1/1
  Product1/1 -> Data Type Conversion1/1

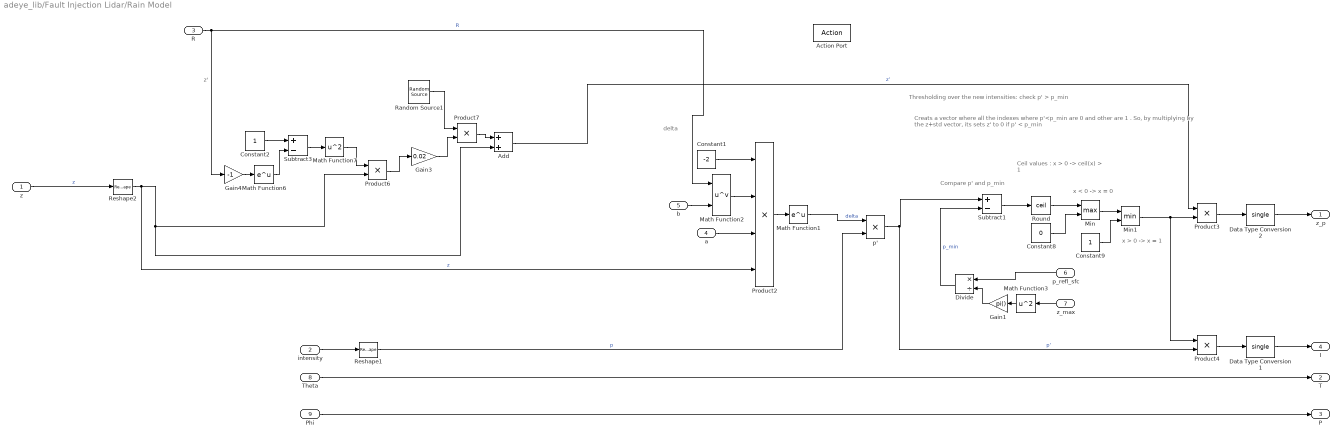
== system adeye_lib/Fault Injection Lidar/Rain Model ==
  note: z'
  note: delta
  note: Thresholding over the new intensities: check p' > p_min
  note: x > 0 -> x = 1
  note: Creats a vector where all the indexes where p'<p_min are 0 and other are 1 .
      | So, by multiplying by the z+std vector, its sets z' to 0 if p' < p_min
  note: Compare p' and p_min
  note: Ceil values :
      | x > 0 -> ceil(x) > 1
  note: x < 0 -> x = 0
  z : Inport
  "intensity " : Inport  Port=2
  R : Inport  Port=3
  "a " : Inport  Port=4
  b : Inport  Port=5
  p_refl_sfc : Inport  Port=6
  z_max : Inport  Port=7
  Theta : Inport  Port=8
  Phi : Inport  Port=9
  Action Port : ActionPort  ActionPortLabel=if(u1 > 1)
  Add : Sum
  Constant1 : Constant  Value=-2
  Constant2 : Constant
  Constant8 : Constant  Value=0
  Constant9 : Constant
  Data Type Conversion1 : DataTypeConversion  OutDataTypeStr=single
  Data Type Conversion2 : DataTypeConversion  OutDataTypeStr=single
  Divide : Product  Inputs=*/
  Gain1 : Gain  Gain=pi()
  Gain3 : Gain  Gain=0.02
  Gain4 : Gain  Gain=-1
  Math Function1 : Math  SaturateOnIntegerOverflow=on
  Math Function2 : Math  Operator=pow  SaturateOnIntegerOverflow=on
  Math Function3 : Math  Operator=square  SaturateOnIntegerOverflow=on
  Math Function6 : Math  SaturateOnIntegerOverflow=on
  Math Function7 : Math  Operator=square  SaturateOnIntegerOverflow=on
  Min : MinMax  Function=max  Inputs=2
  Min1 : MinMax  Inputs=2
  Product2 : Product  Inputs=4
  Product{3..4,6..7} (4 alike) : Product
  Random Source1 : dspsrcs4/Random Source  SrcType=Gaussian  NormMethod=Ziggurat  CltLength=12  MinVal=0  MaxVal=1  MeanVal=0  VarVal=1  RepMode=Not repeatable  rawSeed=1  IsInherit=off  SampMode=Discrete  SampTime=1/(f*p)  SampFrame=p  DataType=Double  OutComplex=Real  OutputFrames=off
  Reshape1 : Reshape  OutputDimensions=[1, 1]
  Reshape2 : Reshape  OutputDimensions=[1, 1]
  Round : Rounding  Operator=ceil
  Subtract1 : Sum  Inputs=+-
  Subtract3 : Sum  Inputs=+-
  p' : Product
  z_p : Outport
  T : Outport  Port=2
  P : Outport  Port=3
  I : Outport  Port=4
  wires:
  z/1 -> Reshape2/1  "z"
  p'/1 -> Product4/2, Subtract1/1  "p'"
  Constant8/1 -> Min/2
  Subtract1/1 -> Round/1
  Divide/1 -> Subtract1/2  "p_min"
  Round/1 -> Min/1
  Min/1 -> Min1/1
  Constant9/1 -> Min1/2
  Min1/1 -> Product4/1, Product3/2
  Math Function1/1 -> p'/1  "delta"
  Math Function2/1 -> Product2/2
  Constant1/1 -> Product2/1
  b/1 -> Math Function2/2
  Product2/1 -> Math Function1/1
  "a "/1 -> Product2/3
  "intensity "/1 -> Reshape1/1
  Data Type Conversion2/1 -> z_p/1
  Reshape2/1 -> Product2/4, Product6/2, Add/2  "z"
  Gain1/1 -> Divide/2
  z_max/1 -> Math Function3/1
  p_refl_sfc/1 -> Divide/1
  Math Function3/1 -> Gain1/1
  Reshape1/1 -> p'/2  "p"
  Product4/1 -> Data Type Conversion1/1
  Product3/1 -> Data Type Conversion2/1
  Theta/1 -> T/1
  Phi/1 -> P/1
  Data Type Conversion1/1 -> I/1
  Add/1 -> Product3/1  "z'"
  Gain4/1 -> Math Function6/1
  Subtract3/1 -> Math Function7/1
  R/1 -> Gain4/1, Math Function2/1  "R"
  Constant2/1 -> Subtract3/1
  Math Function6/1 -> Subtract3/2
  Math Function7/1 -> Product6/1
  Random Source1/1 -> Product7/1
  Product7/1 -> Add/1
  Gain3/1 -> Product7/2
  Product6/1 -> Gain3/1

== system adeye_lib/Fault Injection Listener Camera 1/If Action Subsystem ==
  In1 : Inport
  In2 : Inport  Port=2
  In3 : Inport  Port=3
  In4 : Inport  Port=4
  In5 : Inport  Port=5
  In6 : Inport  Port=6
  In7 : Inport  Port=7
  In8 : Inport  Port=8
  Action Port : ActionPort
  Out1 : Outport
  Out2 : Outport  Port=2
  Out3 : Outport  Port=3
  Out4 : Outport  Port=4
  Out5 : Outport  Port=5
  Out6 : Outport  Port=6
  Out7 : Outport  Port=7
  Out8 : Outport  Port=8
  wires:
  In1/1 -> Out1/1
  In2/1 -> Out2/1
  In3/1 -> Out3/1
  In4/1 -> Out4/1
  In5/1 -> Out5/1
  In6/1 -> Out6/1
  In7/1 -> Out7/1
  In8/1 -> Out8/1

== system adeye_lib/Fault Injection Listener Camera 1/If Action Subsystem1 ==
  In1 : Inport
  In2 : Inport  Port=2
  In3 : Inport  Port=3
  In4 : Inport  Port=4
  In5 : Inport  Port=5
  In6 : Inport  Port=6
  In7 : Inport  Port=7
  In8 : Inport  Port=8
  Action Port : ActionPort
  Out1 : Outport
  Out2 : Outport  Port=2
  Out3 : Outport  Port=3
  Out4 : Outport  Port=4
  Out5 : Outport  Port=5
  Out6 : Outport  Port=6
  Out7 : Outport  Port=7
  Out8 : Outport  Port=8
  wires:
  In1/1 -> Out1/1
  In2/1 -> Out2/1
  In3/1 -> Out3/1
  In4/1 -> Out4/1
  In5/1 -> Out5/1
  In6/1 -> Out6/1
  In7/1 -> Out7/1
  In8/1 -> Out8/1

== system adeye_lib/Fault Injection Listener Camera 2/If Action Subsystem ==
  In1 : Inport
  In2 : Inport  Port=2
  In3 : Inport  Port=3
  In4 : Inport  Port=4
  In5 : Inport  Port=5
  In6 : Inport  Port=6
  In7 : Inport  Port=7
  In8 : Inport  Port=8
  Action Port : ActionPort
  Out1 : Outport
  Out2 : Outport  Port=2
  Out3 : Outport  Port=3
  Out4 : Outport  Port=4
  Out5 : Outport  Port=5
  Out6 : Outport  Port=6
  Out7 : Outport  Port=7
  Out8 : Outport  Port=8
  wires:
  In1/1 -> Out1/1
  In2/1 -> Out2/1
  In3/1 -> Out3/1
  In4/1 -> Out4/1
  In5/1 -> Out5/1
  In6/1 -> Out6/1
  In7/1 -> Out7/1
  In8/1 -> Out8/1

== system adeye_lib/Fault Injection Listener Camera 2/If Action Subsystem1 ==
  In1 : Inport
  In2 : Inport  Port=2
  In3 : Inport  Port=3
  In4 : Inport  Port=4
  In5 : Inport  Port=5
  In6 : Inport  Port=6
  In7 : Inport  Port=7
  In8 : Inport  Port=8
  Action Port : ActionPort
  Out1 : Outport
  Out2 : Outport  Port=2
  Out3 : Outport  Port=3
  Out4 : Outport  Port=4
  Out5 : Outport  Port=5
  Out6 : Outport  Port=6
  Out7 : Outport  Port=7
  Out8 : Outport  Port=8
  wires:
  In1/1 -> Out1/1
  In2/1 -> Out2/1
  In3/1 -> Out3/1
  In4/1 -> Out4/1
  In5/1 -> Out5/1
  In6/1 -> Out6/1
  In7/1 -> Out7/1
  In8/1 -> Out8/1

== system adeye_lib/Fault Injection Listener GNSS/If Action Subsystem ==
  In1 : Inport
  In2 : Inport  Port=2
  Action Port : ActionPort
  Out1 : Outport
  Out2 : Outport  Port=2
  wires:
  In1/1 -> Out1/1
  In2/1 -> Out2/1

== system adeye_lib/Fault Injection Listener GNSS/If Action Subsystem1 ==
  In1 : Inport
  In2 : Inport  Port=2
  Action Port : ActionPort
  Out1 : Outport
  Out2 : Outport  Port=2
  wires:
  In1/1 -> Out1/1
  In2/1 -> Out2/1
